simulink model "excercise1_3tf2"  (R2023b)
settings: Solver=VariableStepAuto  StartTime=0.0  StopTime=3  RelTol=1e-3
undefined symbols (not defined in the file): d, k, m
settings Model: Creator=elliot  LastModifiedBy=elliot

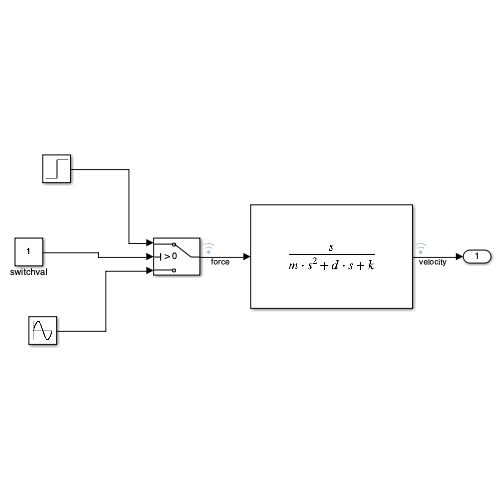
[thumbnail: Simulink's stored preview of the top-level diagram]
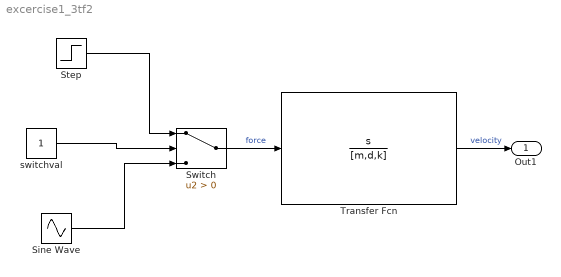
== system excercise1_3tf2 ==
  Sine Wave : Sin  Frequency=10  SampleTime=0
  Step : Step  Time=0  SampleTime=0
  Switch : Switch  Criteria=u2 > Threshold  SaturateOnIntegerOverflow=off  InputSameDT=off
  Transfer Fcn : TransferFcn  Numerator=[1,0]  Denominator=[m,d,k]
  switchval : Constant
  Out1 : Outport
  wires:
  switchval/1 -> Switch/2
  Switch/1 -> Transfer Fcn/1  "force"
  Transfer Fcn/1 -> Out1/1  "velocity"
  Step/1 -> Switch/1
  Sine Wave/1 -> Switch/3
